simulink model "reaction_pendulum_23b_anders"  (R2023b)
settings: Solver=FixedStepDiscrete  StartTime=0.0  StopTime=10  FixedStep=h  RelTol=1e-3  EnableMultiTasking=on
PreLoadFcn:
  | warning('off','MATLAB:dispatcher:InexactMatch');
InitFcn:
  | hwinit
  | LQR_gain
model workspace (MAT data in the model file):
  square_freq = 0.5
values from neighbouring files (symbols this model uses):
  F = A22-L*A12    [Reduced_observer.m]
  G = A21-L*A11+F*L    [Reduced_observer.m]
  h = 0.05    [hwinit.m]
  H = B2-L*B1    [Reduced_observer.m]
  K_LQR = lqr(A,B,Q,R)    [LQR_gain.m]
  L = 10    [LQR_gain.m]    (also in Reduced_observer.m = place(A22',A12',pole)')
undefined symbols (not defined in the file or in its folder): DiscIntNeverNeededParam
libraries: dspsrcs4 x1
settings Model: ExtModeTrigDuration=100000  Creator=user  LastModifiedBy=india
settings DataIOCC: SaveFormat=Array  SignalLoggingSaveFormat=ModelDataLogs  SaveOutput=off  SignalLogging=off  DSMLogging=off  SaveTime=off  ReturnWorkspaceOutputs=off
settings OptimizationCC: ExpressionDepthLimit=2147483647  LifeSpan=inf
settings DebuggingCC: UnderspecifiedInitializationDetection=Classic  MergeDetectMultiDrivingBlocksExec=none  SolverPrmCheckMsg=warning  FcnCallInpInsideContextMsg=warning  UnconnectedInputMsg=warning  UnconnectedOutputMsg=warning  UnconnectedLineMsg=warning  StateNameClashWarn=warning  SFUnexpectedBacktrackingDiag=warning  SFNoUnconditionalDefaultTransitionDiag=warning  SFExecutionAtInitializationDiag=none  ArithmeticOperatorsInVariantConditions=warning
settings HardwareCC: ProdBitPerPointer=32  ProdBitPerSizeT=32  ProdBitPerPtrDiffT=32  ProdLargestAtomicFloat=None  ProdIntDivRoundTo=Undefined  ProdEndianess=Unspecified  ProdWordSize=32  ProdHWDeviceType=32-bit Generic
settings ModelReferenceCC: EnableRefExpFcnMdlSchedulingChecks=on  PropagateSignalLabelsOutOfModel=off
settings SFSimCC: SimUseLocalCustomCode=off  CustomCodeUndefinedFunction=UseInterfaceOnly
settings RTWCC: Description=rpend RTDAC/USB2 (Visual C/C++)  SystemTargetFile=rtcon_rpend_usb2.tlc  TemplateMakefile=rtcon_rpend_vc_usb2_x64.tmf  RTWUseLocalCustomCode=off  DLArmComputeVersion=19.05
settings CodeAppCC: StateflowObjectComments=on
settings STFCustomTargetCC: TargetLangStandard=C89/C90 (ANSI)  ModelReferenceCompliant=off  CombineOutputUpdateFcns=on  MatFileLogging=on  SystemTargetFile=rtcon_rpend_usb2.tlc
settings GRTTargetCC: TargetLangStandard=C89/C90 (ANSI)  ModelReferenceCompliant=off  ParMdlRefBuildCompliant=off  CompOptLevelCompliant=off  ConcurrentExecutionCompliant=off  CPPClassGenCompliant=off  UseToolchainInfoCompliant=off  ExtMode=on  ExtModeMexFile=rtcon_ext_comm
settings ConfigComp: CovMetricSettings=dw  CovSaveCumulativeToWorkspaceVar=on  CovSaveSingleToWorkspaceVar=on  CovExternalEMLEnable=off  CovSFcnEnable=off

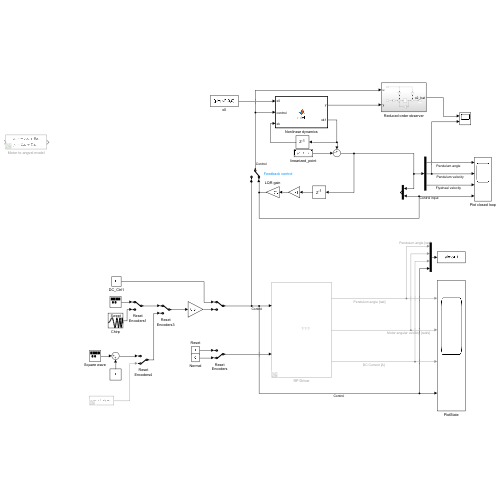
[thumbnail: Simulink's stored preview of the top-level diagram]
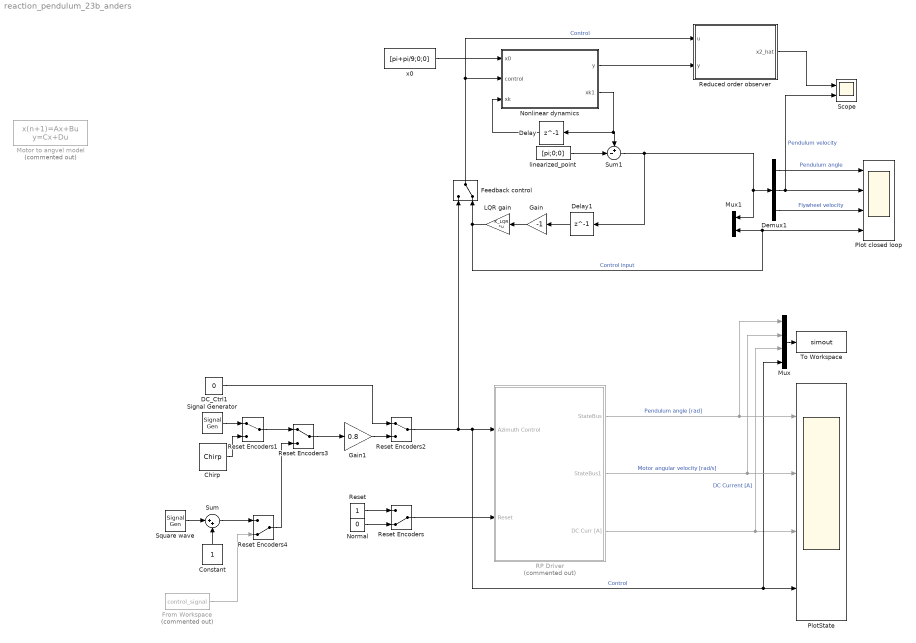
== system reaction_pendulum_23b_anders ==
  Chirp : dspsrcs4/Chirp  sweep=Swept cosine  mode=Unidirectional  f0=0.1  f1=0.8  t1=30  Tsweep=30  phase=0  Ts=h  spf=1  datatype=Double  OutputFrames=off
  Constant : Constant
  DC_Ctrl1 : Constant  Value=0
  Delay : Delay  DelayLength=1
  Delay1 : Delay  DelayLength=1
  Demux1 : Demux  Outputs=3
  Feedback control : ManualSwitch  CurrentSetting=0
  From Workspace : FromWorkspace  Commented=on  VariableName=control_signal  SampleTime=-1
  Gain : Gain  Gain=-1
  Gain1 : Gain  Gain=0.8
  LQR gain : Gain  Gain=K_LQR  Multiplication=Matrix(K*u)
  Motor to angvel model : DiscreteStateSpace  Commented=on  A=exp(-0.9403*0.05)  B=402.0068*0.05  D=0  SampleTime=-1
  Mux : Mux
  Mux1 : Mux  Inputs=2
  Nonlinear dynamics : MATLAB Function  TreatAsAtomicUnit=on
  Normal : Constant  Value=0
  Plot closed loop : Scope  NumInputPorts=4
  PlotState : Scope  NumInputPorts=4
  RP Driver : Subsystem  Commented=on
      mask Display: image(imread('rwp.JPG'))
  Reduced order observer : Subsystem
  Reset : Constant
  Reset Encoders : ManualSwitch  CurrentSetting=0
  Reset Encoders1 : ManualSwitch
  Reset Encoders2 : ManualSwitch
  Reset Encoders3 : ManualSwitch
  Reset Encoders4 : ManualSwitch  CurrentSetting=0
  Scope : Scope  NumInputPorts=2
  Signal Generator : SignalGenerator  Frequency=0.2
  Square wave : SignalGenerator  WaveForm=square  Frequency=0.1
  Sum : Sum  Inputs=|++
  Sum1 : Sum  Inputs=+-|
  To Workspace : ToWorkspace  VariableName=simout  SaveFormat=Structure With Time  SampleTime=-1
      settings: Save2DSignal=2-D array (concatenate along first dimension)
  linearized_point : Constant  Value=[pi;0;0]
  x0 : Constant  Value=[pi+pi/9;0;0]
  wires:
  Normal/1 -> Reset Encoders/2
  Reset/1 -> Reset Encoders/1
  Reset Encoders/1 -> RP Driver/2(Reset)
  RP Driver/3(DC Curr [A]) -> Mux/3, PlotState/3  "DC Current [A]"
  Reset Encoders2/1 -> RP Driver/1(Azimuth Control), Mux/4, PlotState/4, Feedback control/1  "Control"
  DC_Ctrl1/1 -> Reset Encoders2/1
  RP Driver/2(StateBus1) -> Mux/2, PlotState/2  "Motor angular velocity [rad/s]"
  Gain1/1 -> Reset Encoders2/2
  RP Driver/1(StateBus) -> Mux/1, PlotState/1  "Pendulum angle [rad]"
  Mux/1 -> To Workspace/1
  Signal Generator/1 -> Reset Encoders1/1
  Chirp/1 -> Reset Encoders1/2
  Square wave/1 -> Sum/1
  Constant/1 -> Sum/2
  Reset Encoders1/1 -> Reset Encoders3/1
  Reset Encoders3/1 -> Gain1/1
  Reset Encoders4/1 -> Reset Encoders3/2
  Sum/1 -> Reset Encoders4/1
  From Workspace/1 -> Reset Encoders4/2
  Nonlinear dynamics/2(xk1) -> Sum1/1, Delay/1
  Delay/1 -> Nonlinear dynamics/3(xk)
  x0/1 -> Nonlinear dynamics/1(x0)
  Feedback control/1 -> Reduced order observer/1(u), Nonlinear dynamics/2(control)  "Control"
  LQR gain/1 -> Mux1/2, Plot closed loop/4, Feedback control/2  "Control input"
  Sum1/1 -> Delay1/1, Mux1/1, Demux1/1
  Gain/1 -> LQR gain/1
  Delay1/1 -> Gain/1
  Demux1/3 -> Plot closed loop/3  "Flywheel velocity"
  Demux1/2 -> Scope/2, Plot closed loop/2  "Pendulum velocity"
  Demux1/1 -> Plot closed loop/1  "Pendulum angle"
  linearized_point/1 -> Sum1/2
  Nonlinear dynamics/1(y) -> Reduced order observer/2(y)
  Reduced order observer/1(x2_hat) -> Scope/1

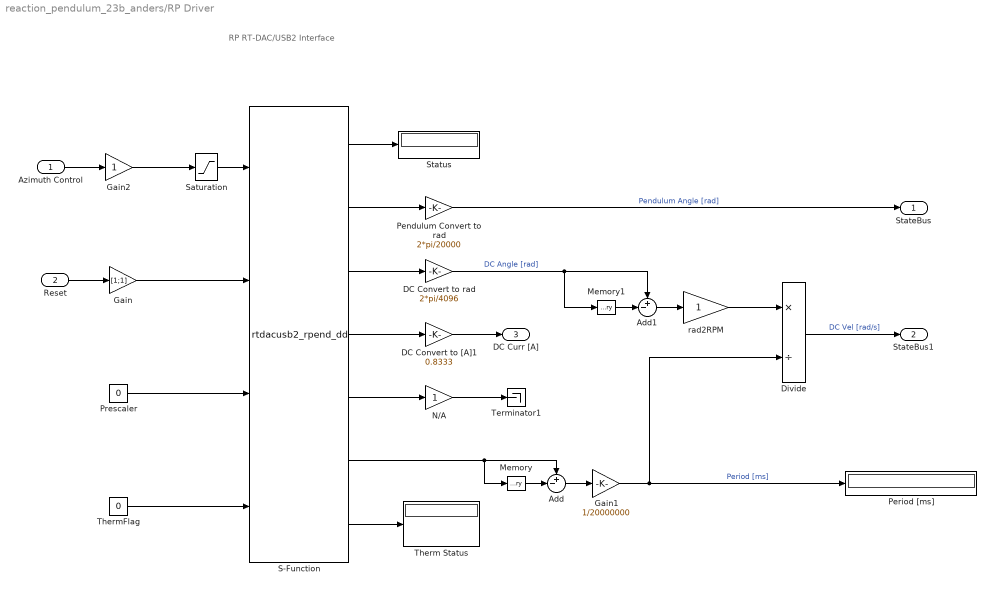
== system reaction_pendulum_23b_anders/RP Driver ==
  note: RP RT-DAC/USB2
      | Interface
  Azimuth Control : Inport
  Reset : Inport  Port=2
  Add : Sum  Inputs=+-|
  Add1 : Sum  Inputs=+-|
  DC Convert to [A]1 : Gain  Gain=0.8333  SaturateOnIntegerOverflow=on  OutDataTypeStr=Inherit: Same as input  ParamDataTypeStr=Inherit: Same as input
  DC Convert to rad : Gain  Gain=2*pi/4096  SaturateOnIntegerOverflow=on  OutDataTypeStr=Inherit: Same as input  ParamDataTypeStr=Inherit: Same as input
  Divide : Product  Inputs=*/
  Gain : Gain  Gain=[1;1]
  Gain1 : Gain  Gain=1/20000000
  Gain2 : Gain
  Memory : Memory
  Memory1 : Memory
  N/A : Gain  SaturateOnIntegerOverflow=on  OutDataTypeStr=Inherit: Same as input  ParamDataTypeStr=Inherit: Same as input
  Pendulum Convert to rad : Gain  Gain=2*pi/20000  SaturateOnIntegerOverflow=on  OutDataTypeStr=Inherit: Same as input  ParamDataTypeStr=Inherit: Same as input
  Period [ms] : Display
  Prescaler : Constant  Value=0
  S-Function : S-Function  FunctionName=rtdacusb2_rpend_dd  Parameters=1, h  SFunctionDeploymentMode=off  EnableBusSupport=off
  Saturation : Saturate  UpperLimit=1  LowerLimit=-1
  Status : Display
  Terminator1 : Terminator
  Therm Status : Display
  ThermFlag : Constant  Value=0
  rad2RPM : Gain  SaturateOnIntegerOverflow=on  OutDataTypeStr=Inherit: Same as input  ParamDataTypeStr=Inherit: Same as input
  StateBus : Outport  VectorParamsAs1DForOutWhenUnconnected=off
  StateBus1 : Outport  Port=2  VectorParamsAs1DForOutWhenUnconnected=off
  DC Curr [A] : Outport  Port=3  VectorParamsAs1DForOutWhenUnconnected=off
  wires:
  S-Function/7 -> Therm Status/1
  S-Function/5 -> N/A/1
  S-Function/4 -> DC Convert to [A]1/1
  ThermFlag/1 -> S-Function/4
  Prescaler/1 -> S-Function/3
  Gain/1 -> S-Function/2
  DC Convert to [A]1/1 -> DC Curr [A]/1
  Divide/1 -> StateBus1/1  "DC Vel [rad/s]"
  rad2RPM/1 -> Divide/1
  Add1/1 -> rad2RPM/1
  Memory1/1 -> Add1/2
  N/A/1 -> Terminator1/1
  S-Function/6 -> Add/1, Memory/1
  Gain2/1 -> Saturation/1
  Gain1/1 -> Period [ms]/1, Divide/2  "Period [ms]"
  Add/1 -> Gain1/1
  Memory/1 -> Add/2
  DC Convert to rad/1 -> Add1/1, Memory1/1  "DC Angle [rad]"
  S-Function/3 -> DC Convert to rad/1
  Pendulum Convert to rad/1 -> StateBus/1  "Pendulum Angle [rad]"
  S-Function/2 -> Pendulum Convert to rad/1
  S-Function/1 -> Status/1
  Saturation/1 -> S-Function/1
  Reset/1 -> Gain/1
  Azimuth Control/1 -> Gain2/1

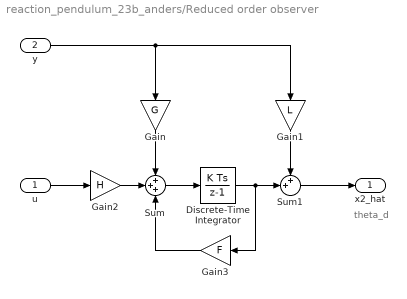
== system reaction_pendulum_23b_anders/Reduced order observer ==
  note: theta_d
  u : Inport
  y : Inport  Port=2
  Discrete-Time Integrator : DiscreteIntegrator  SampleTime=-1  ICPrevOutput=DiscIntNeverNeededParam  ICPrevScaledInput=DiscIntNeverNeededParam
  Gain : Gain  Gain=G
  Gain1 : Gain  Gain=L
  Gain2 : Gain  Gain=H
  Gain3 : Gain  Gain=F
  Sum : Sum  Inputs=+++
  Sum1 : Sum  Inputs=++|
  x2_hat : Outport
  wires:
  u/1 -> Gain2/1
  Gain2/1 -> Sum/2
  Gain/1 -> Sum/1
  Sum/1 -> Discrete-Time Integrator/1
  Gain1/1 -> Sum1/1
  Discrete-Time Integrator/1 -> Gain3/1, Sum1/2
  Gain3/1 -> Sum/3
  Sum1/1 -> x2_hat/1
  y/1 -> Gain1/1, Gain/1

== matlab function reaction_pendulum_23b_anders/Nonlinear dynamics ==
  data: x0 input; y output; control input; xk input size=[3,1]; xk1 output size=[3,1]; h parameter
function [y, xk1] = nlrk4(x0, control, xk, h)
    persistent initialized

    if isempty(initialized)
        xk = x0;
        initialized = true;
    end

    function dx = nlf(t,x,u)
    
        % Define constants
        K1 = 10.6608;
        K2 = 0.0487;
        K3 = 0.1031;
        K4 = 404.3827;
        K5 = 0.9442;
        K6 = 1.7125;
        K_tau = 0.0107;
        
        % System equations
        theta = x(1);
        theta_dot = x(2);
        omega = x(3);
        theta_ddot = -K1*sin(theta)-K2*theta_dot-K3*sign(theta_dot)-K_tau*(K4*u-K5*omega-K6*sign(omega));
        omega_dot = K4*u-K5*omega-K6*sign(omega);
        dx = [theta_dot; theta_ddot; omega_dot];
    end

    % Executes one timestep of the RK4 algorithm
    k1 = nlf(0, xk, control);
    k2 = nlf(0 + h/2, xk + h/2*k1, control);
    k3 = nlf(0 + h/2, xk + h/2*k2, control);
    k4 = nlf(0 + h, xk + h*k3, control);
    xk1 = xk + h/6*(k1 + 2*k2 + 2*k3 + k4);
    % Take out states of interest
    y = [xk(1); xk(3)];
end
